simulink model "Control_test"  (R2014b)
settings: Solver=FixedStepDiscrete  StartTime=0.0  StopTime=Inf  FixedStep=0.001  RelTol=1e-3
PostLoadFcn:
  | , if any(exist('dsrtsu_mdlpostloadfcn', 'file') == [2, 3, 6]), try dsrtsu_mdlpostloadfcn('Execute', bdroot); catch fprintf('Error in PostLoadFcn (dsrtsu_mdlpostloadfcn) for model "%s":\n %s\n', bdroot, lasterr); end, end,
undefined symbols (not defined in the file or in its folder): dtLocal, slcm
libraries: rtican x163, simulink x14
(part 6 of 34)

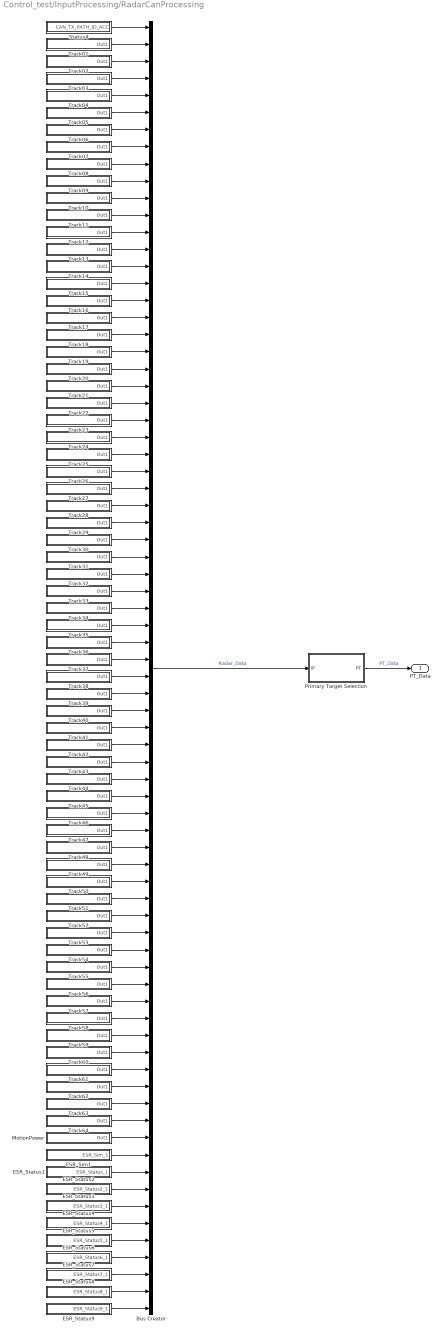
== system Control_test/InputProcessing/RadarCanProcessing ==
  Bus Creator : BusCreator  Inputs=76
  ESR_Sim1 : Subsystem
  ESR_Status1 : Subsystem
  ESR_Status2 : Subsystem
  ESR_Status3 : Subsystem
  ESR_Status4 : Subsystem
  ESR_Status5 : Subsystem
  ESR_Status6 : Subsystem
  ESR_Status7 : Subsystem
  ESR_Status8 : Subsystem
  ESR_Status9 : Subsystem
  MotionPower : Subsystem
  Primary Target Selection : Subsystem
  Status4 : Subsystem
  Track01 : Subsystem
  Track02 : Subsystem
  Track03 : Subsystem
  Track04 : Subsystem
  Track05 : Subsystem
  Track06 : Subsystem
  Track07 : Subsystem
  Track08 : Subsystem
  Track09 : Subsystem
  Track10 : Subsystem
  Track11 : Subsystem
  Track12 : Subsystem
  Track13 : Subsystem
  Track14 : Subsystem
  Track15 : Subsystem
  Track16 : Subsystem
  Track17 : Subsystem
  Track18 : Subsystem
  Track19 : Subsystem
  Track20 : Subsystem
  Track21 : Subsystem
  Track22 : Subsystem
  Track23 : Subsystem
  Track24 : Subsystem
  Track25 : Subsystem
  Track26 : Subsystem
  Track27 : Subsystem
  Track28 : Subsystem
  Track29 : Subsystem
  Track30 : Subsystem
  Track31 : Subsystem
  Track32 : Subsystem
  Track33 : Subsystem
  Track34 : Subsystem
  Track35 : Subsystem
  Track36 : Subsystem
  Track37 : Subsystem
  Track38 : Subsystem
  Track39 : Subsystem
  Track40 : Subsystem
  Track41 : Subsystem
  Track42 : Subsystem
  Track43 : Subsystem
  Track44 : Subsystem
  Track45 : Subsystem
  Track46 : Subsystem
  Track47 : Subsystem
  Track48 : Subsystem
  Track49 : Subsystem
  Track50 : Subsystem
  Track51 : Subsystem
  Track52 : Subsystem
  Track53 : Subsystem
  Track54 : Subsystem
  Track55 : Subsystem
  Track56 : Subsystem
  Track57 : Subsystem
  Track58 : Subsystem
  Track59 : Subsystem
  Track60 : Subsystem
  Track61 : Subsystem
  Track62 : Subsystem
  Track63 : Subsystem
  Track64 : Subsystem
  PT_Data : Outport
  wires:
  Status4/1(CAN_TX_PATH_ID_ACC) -> Bus Creator/1
  Track01/1(Out1) -> Bus Creator/2
  Track02/1(Out1) -> Bus Creator/3
  Track03/1(Out1) -> Bus Creator/4
  Track04/1(Out1) -> Bus Creator/5
  Track05/1(Out1) -> Bus Creator/6
  Track06/1(Out1) -> Bus Creator/7
  Track07/1(Out1) -> Bus Creator/8
  Track08/1(Out1) -> Bus Creator/9
  Track09/1(Out1) -> Bus Creator/10
  Track10/1(Out1) -> Bus Creator/11
  Track11/1(Out1) -> Bus Creator/12
  Track12/1(Out1) -> Bus Creator/13
  Track13/1(Out1) -> Bus Creator/14
  Track14/1(Out1) -> Bus Creator/15
  Track15/1(Out1) -> Bus Creator/16
  Track16/1(Out1) -> Bus Creator/17
  Track17/1(Out1) -> Bus Creator/18
  Track18/1(Out1) -> Bus Creator/19
  Track19/1(Out1) -> Bus Creator/20
  Track20/1(Out1) -> Bus Creator/21
  Track21/1(Out1) -> Bus Creator/22
  Track22/1(Out1) -> Bus Creator/23
  Track23/1(Out1) -> Bus Creator/24
  Track24/1(Out1) -> Bus Creator/25
  Track25/1(Out1) -> Bus Creator/26
  Track26/1(Out1) -> Bus Creator/27
  Track27/1(Out1) -> Bus Creator/28
  Track28/1(Out1) -> Bus Creator/29
  Track29/1(Out1) -> Bus Creator/30
  Track30/1(Out1) -> Bus Creator/31
  Track31/1(Out1) -> Bus Creator/32
  Track32/1(Out1) -> Bus Creator/33
  Track33/1(Out1) -> Bus Creator/34
  Track34/1(Out1) -> Bus Creator/35
  Track35/1(Out1) -> Bus Creator/36
  Track36/1(Out1) -> Bus Creator/37
  Track37/1(Out1) -> Bus Creator/38
  Track38/1(Out1) -> Bus Creator/39
  Track39/1(Out1) -> Bus Creator/40
  Track40/1(Out1) -> Bus Creator/41
  Track41/1(Out1) -> Bus Creator/42
  Track42/1(Out1) -> Bus Creator/43
  Track43/1(Out1) -> Bus Creator/44
  Track44/1(Out1) -> Bus Creator/45
  Track45/1(Out1) -> Bus Creator/46
  Track46/1(Out1) -> Bus Creator/47
  Track47/1(Out1) -> Bus Creator/48
  Track48/1(Out1) -> Bus Creator/49
  Track49/1(Out1) -> Bus Creator/50
  Track50/1(Out1) -> Bus Creator/51
  Track51/1(Out1) -> Bus Creator/52
  Track52/1(Out1) -> Bus Creator/53
  Track53/1(Out1) -> Bus Creator/54
  Track54/1(Out1) -> Bus Creator/55
  Track55/1(Out1) -> Bus Creator/56
  Track56/1(Out1) -> Bus Creator/57
  Track57/1(Out1) -> Bus Creator/58
  Track58/1(Out1) -> Bus Creator/59
  Track59/1(Out1) -> Bus Creator/60
  Track60/1(Out1) -> Bus Creator/61
  Track61/1(Out1) -> Bus Creator/62
  Track62/1(Out1) -> Bus Creator/63
  Track63/1(Out1) -> Bus Creator/64
  Track64/1(Out1) -> Bus Creator/65
  Bus Creator/1 -> Primary Target Selection/1(IP)  "Radar_Data"
  MotionPower/1(Out1) -> Bus Creator/66
  Primary Target Selection/1(PT) -> PT_Data/1  "PT_Data"
  ESR_Sim1/1(ESR_Sim_1) -> Bus Creator/67
  ESR_Status1/1(ESR_Status_1) -> Bus Creator/68
  ESR_Status2/1(ESR_Status2_1) -> Bus Creator/69
  ESR_Status3/1(ESR_Status3_1) -> Bus Creator/70
  ESR_Status4/1(ESR_Status4_1) -> Bus Creator/71
  ESR_Status5/1(ESR_Status5_1) -> Bus Creator/72
  ESR_Status6/1(ESR_Status6_1) -> Bus Creator/73
  ESR_Status7/1(ESR_Status7_1) -> Bus Creator/74
  ESR_Status8/1(ESR_Status8_1) -> Bus Creator/75
  ESR_Status9/1(ESR_Status9_1) -> Bus Creator/76

== system Control_test/InputProcessing/SensorFusion ==
  Bus Creator : BusCreator  Inputs=2
  Bus Creator1 : BusCreator  Inputs=2
  Bus Creator2 : BusCreator  Inputs=2
  Bus Creator3 : BusCreator  Inputs=3
  PTLeft_Data : rtican/RTICAN Receive (RX)   Reserved1=[]  Reserved2=[]  Reserved3=[]  Reserved4=[]  SfcnMessage=[]  Msg_Struct=[]  BoardTypeNo=[]  BoardNo=[]  ChannelNo=[]  Parameters=[]  DialogFcn=[]  UnitName=[]  Revision=[]  UnitValues=[]  DSProperties=struct('RTI',struct('Version',uint32(5),'BlockType',struct('isSLSource',uint8(1),'isSLSink',uint8(1),'isHWSource',uint8(0),'isHWSink',uint8(0),'isSetup',uint8(0),'isInline',uint8(1),'isNonInline',uint8(0),'isInterrupt',uint8(0),'isChannelwise',uint8(0)),'IOBoardType','RTICAN','UnitType','MESSAGE','Identifier','RX','DialogType','MSVC','BlockSet','RTICAN','SlaveProcessor','CAN'))  RTIBlockInterface=struct('OutputPortsWidth',int32([1 1]),'OutputPortsActive',[1 1],'OutputPortsName',{{'PTLeft_RelDist','PTLeft_RelSpeed'}},'OutputPortsDataType',{{'SS_DOUBLE','SS_DOUBLE'}},'OutputPortsLabel',{{'PTLeft_RelDist','PTLeft_RelSpeed'}},'OutputPortsLabelMode','ON','InputPortsWidth',int32(0),'InputPortsActive',0,'DialogFcn','rtican_message_interface_gui','BlockDisplay',{{'','center'}},'IconTransparency','on','ParameterTunableNames',{{}},'InitLevel',3,'BlockName',struct('Token',{{'PTLeft_Data'}}),'SampleTime',{{0.01}},'TriggerPort',{{'none'}},'EnablePort',{{'none'}})  RTIBlockParameters=struct('BoardTypeNo',{{1,'OFF',[]}},'BoardNo',{{2,'ON',[1 16]}},'ChannelNo',{{2,'ON',[1 2]}},'Parameters',{{struct('DataFileSupport',struct('DataFileSelectedMaster',1,'DataFileSelectedLocal',1,'DataFileName',['c:\users\mpc\documents\github\mpc-car\controller\dbcfiles\esr_dv3_64tgt.dbc|c:\users\mpc\dropbox\hyundai car setup\01_dbc_files\sensorfusion.dbc|'],'DataFileDate',['15-Dec-2015 14:58:47'],'SelectedFile',['..\..\..\..\..\..\dropbox\hyundai car setup\01_dbc_files\sensorfusion.dbc'],'InterfaceFcn','rtican_dbc_file_parser'),'Options',struct('StatusSelected',0,'TimeSelected',0,'DeltaTimeSelected',0,'BytePortSelected',0,'MessageLengthSelected',0,'TriggerPort',struct('Selected',0,'TriggerType',0),'UserCoding',struct('Selected',0,'InterfaceFile','UserDecodingFile','FcnName','UserDecodeFcn','InportSelected',0,'InportWidth',1,'OutportSelected',0,'OutportWidth',1),'EnablePortSelected',0,'SignalOnPortnameSelected',1,'UseRXService',0),'Message',struct('MsgOnBlocknameSelected',1,'MsgName','PTLeft_Data','MsgIdFormat',0,'MsgId',1585,'MsgLength',8,'NumSignals',2,'SampleTime',0.01,'Signal',struct('SgnName',{'PTLeft_RelDist','PTLeft_RelSpeed'},'SgnStartBit',{0,16},'SgnLength',{16,16},'SgnType',{0,0},'ModeValue',{-1,-1},'DataType',{1,1},'ByteLayout',{0,0},'Factor',{0.01,0.01},'Offset',{0,0},'SgnComment',{{''},{''}},'SgnUnit',{'m','m/s'},'Min',{-327.68,-327.68},'Max',{327.67,327.67},'SLDataType',{'SS_DOUBLE','SS_DOUBLE'}),'MsgIdNumFormat',0,'MsgComment',{{''}}),'Version',1.2,'general',struct('isFromLib',0)),'OFF',[]}},'GroupId',{{struct('Group',{{'RTICAN'}},'No',4,'Behavior',{{'NAMECHANGE'}},'BlockType',{{'SINK'}},'NameChangeFlag',0),'OFF',[]}},'SFcnRTICANMessage',{{struct('MsgType','RX','SFcnPortType','Scalar','MsgName','PTLeft_Data','MsgIdFormat','STD','MsgId',1585,'MsgLength',8,'NumSignals',2,'SampleTime',0.01,'Signal',struct('SgnName',{'PTLeft_RelDist','PTLeft_RelSpeed'},'SgnStartBit',{0,16},'SgnLength',{16,16},'SgnType',{'standard','standard'},'ModeValue',{-1,-1},'DataType',{['signed int'],['signed int']},'ByteLayout',{['little endian'],['little endian']},'Factor',{0.01,0.01},'Offset',{0,0},'SLDataType',{'SS_DOUBLE','SS_DOUBLE'}),'StatusSelected','no','TimeSelected','no','DeltaTimeSelected','no','BytePortSelected','no','MessageLengthSelected','no','TriggerPort',struct('Selected','no','TriggerType',0),'UserCoding',struct('Selected','no','InterfaceFile','UserDecodingFile','FcnName','UserDecodeFcn','InportSelected','no','InportWidth',1,'OutportSelected','no','OutportWidth',1),'EnablePortSelected','no','UseRXService','no','BoardType','DS1','BoardNo',2,'ControllerNo',2),'OFF',[]}},'TLCFileName',{{'rtican_rx_message','OFF',[]}})  RTISFcnParameters=struct('SFcnRTICANMessage','struct','TLCFileName','char')  RTIBlockParaDefault=struct('BoardTypeNo',4302,'BoardNo',1,'ChannelNo',1,'Parameters',struct('DataFileSupport',struct('DataFileSelectedMaster',0,'DataFileSelectedLocal',0,'DataFileName','','DataFileDate','','SelectedFile',['<no file selected>']),'Options',struct('StatusSelected',1,'TimeSelected',1,'DeltaTimeSelected',1,'BytePortSelected',0,'MessageLengthSelected',0,'TriggerPort',struct('Selected',0,'TriggerType','rising'),'UserCoding',struct('Selected',0,'InterfaceFile','UserDecodingFile','FcnName','UserDecodeFcn','InportSelected',0,'InportWidth',1,'OutportSelected',0,'OutportWidth',1),'EnablePortSelected',0,'SignalOnPortnameSelected',1,'UseRXService',0),'Message',struct('MsgOnBlocknameSelected',0,'MsgName',['RX Message'],'MsgIdFormat',0,'MsgId',100,'MsgLength',8,'NumSignals',1,'SampleTime',-1,'Signal',struct('SgnName',['RX signal'],'SgnStartBit',0,'SgnLength',8,'SgnType',0,'ModeValue',-1,'DataType',0,'SLDataType','SS_DOUBLE','ByteLayout',0,'Factor',1,'Offset',0,'Min',0,'Max',255,'SgnComment',{{}},'SgnUnit',''),'MsgIdNumFormat',0,'MsgComment',{{''}}),'Version',1.2,'general',struct('isFromLib',1)),'GroupId',struct('Group',{{'RTICAN'}},'No',1,'Behavior',{{'NAMECHANGE'}},'BlockType',{{'SINK'}},'NameChangeFlag',0),'SFcnRTICANMessage',struct('MsgType','RX','MsgName',['RX Message'],'MsgIdFormat','STD','MsgId',100,'MsgLength',8,'NumSignals',1,'SampleTime',-1,'Signal',struct('SgnName',['RX signal'],'SgnStartBit',0,'SgnLength',8,'SgnType','standard','ModeValue',-1,'DataType',['unsigned int'],'ByteLayout',['little endian'],'SLDataType','SS_DOUBLE','Factor',1,'Offset',0),'StatusSelected','yes','TimeSelected','yes','DeltaTimeSelected','yes','BytePortSelected','no','MessageLengthSelected','no','EnablePortSelected','no','UserCoding',struct('Selected','no','InterfaceFile','UserDecodingFile','FcnName','UserDecodeFcn','InportSelected','no','InportWidth',1,'OutportSelected','no','OutportWidth',1),'TriggerPort',struct('Selected','no','TriggerType','rising'),'UseRXService','no','BoardType','DS4302','BoardNo',1,'ControllerNo',1,'SFcnPortType','Scalar'),'TLCFileName','rtican_rx_message')
      settings: AttributesFormatString=Group Id: RTICAN4\n
  PTRight_Data : rtican/RTICAN Receive (RX)   Reserved1=[]  Reserved2=[]  Reserved3=[]  Reserved4=[]  SfcnMessage=[]  Msg_Struct=[]  BoardTypeNo=[]  BoardNo=[]  ChannelNo=[]  Parameters=[]  DialogFcn=[]  UnitName=[]  Revision=[]  UnitValues=[]  DSProperties=struct('RTI',struct('Version',uint32(5),'BlockType',struct('isSLSource',uint8(1),'isSLSink',uint8(1),'isHWSource',uint8(0),'isHWSink',uint8(0),'isSetup',uint8(0),'isInline',uint8(1),'isNonInline',uint8(0),'isInterrupt',uint8(0),'isChannelwise',uint8(0)),'IOBoardType','RTICAN','UnitType','MESSAGE','Identifier','RX','DialogType','MSVC','BlockSet','RTICAN','SlaveProcessor','CAN'))  RTIBlockInterface=struct('OutputPortsWidth',int32([1 1]),'OutputPortsActive',[1 1],'OutputPortsName',{{'PTRight_RelDist','PTRight_RelSpeed'}},'OutputPortsDataType',{{'SS_DOUBLE','SS_DOUBLE'}},'OutputPortsLabel',{{'PTRight_RelDist','PTRight_RelSpeed'}},'OutputPortsLabelMode','ON','InputPortsWidth',int32(0),'InputPortsActive',0,'DialogFcn','rtican_message_interface_gui','BlockDisplay',{{'','center'}},'IconTransparency','on','ParameterTunableNames',{{}},'InitLevel',3,'BlockName',struct('Token',{{'PTRight_Data'}}),'SampleTime',{{0.01}},'TriggerPort',{{'none'}},'EnablePort',{{'none'}})  RTIBlockParameters=struct('BoardTypeNo',{{1,'OFF',[]}},'BoardNo',{{2,'ON',[1 16]}},'ChannelNo',{{2,'ON',[1 2]}},'Parameters',{{struct('DataFileSupport',struct('DataFileSelectedMaster',1,'DataFileSelectedLocal',1,'DataFileName',['c:\users\mpc\documents\github\mpc-car\controller\dbcfiles\esr_dv3_64tgt.dbc|c:\users\mpc\dropbox\hyundai car setup\01_dbc_files\sensorfusion.dbc|'],'DataFileDate',['15-Dec-2015 14:58:47'],'SelectedFile',['..\..\..\..\..\..\dropbox\hyundai car setup\01_dbc_files\sensorfusion.dbc'],'InterfaceFcn','rtican_dbc_file_parser'),'Options',struct('StatusSelected',0,'TimeSelected',0,'DeltaTimeSelected',0,'BytePortSelected',0,'MessageLengthSelected',0,'TriggerPort',struct('Selected',0,'TriggerType',0),'UserCoding',struct('Selected',0,'InterfaceFile','UserDecodingFile','FcnName','UserDecodeFcn','InportSelected',0,'InportWidth',1,'OutportSelected',0,'OutportWidth',1),'EnablePortSelected',0,'SignalOnPortnameSelected',1,'UseRXService',0),'Message',struct('MsgOnBlocknameSelected',1,'MsgName','PTRight_Data','MsgIdFormat',0,'MsgId',1586,'MsgLength',8,'NumSignals',2,'SampleTime',0.01,'Signal',struct('SgnName',{'PTRight_RelDist','PTRight_RelSpeed'},'SgnStartBit',{0,16},'SgnLength',{16,16},'SgnType',{0,0},'ModeValue',{-1,-1},'DataType',{1,1},'ByteLayout',{0,0},'Factor',{0.01,0.01},'Offset',{0,0},'SgnComment',{{''},{''}},'SgnUnit',{'m','m/s'},'Min',{-327.68,-327.68},'Max',{327.67,327.67},'SLDataType',{'SS_DOUBLE','SS_DOUBLE'}),'MsgIdNumFormat',0,'MsgComment',{{''}}),'Version',1.2,'general',struct('isFromLib',0)),'OFF',[]}},'GroupId',{{struct('Group',{{'RTICAN'}},'No',4,'Behavior',{{'NAMECHANGE'}},'BlockType',{{'SINK'}},'NameChangeFlag',0),'OFF',[]}},'SFcnRTICANMessage',{{struct('MsgType','RX','SFcnPortType','Scalar','MsgName','PTRight_Data','MsgIdFormat','STD','MsgId',1586,'MsgLength',8,'NumSignals',2,'SampleTime',0.01,'Signal',struct('SgnName',{'PTRight_RelDist','PTRight_RelSpeed'},'SgnStartBit',{0,16},'SgnLength',{16,16},'SgnType',{'standard','standard'},'ModeValue',{-1,-1},'DataType',{['signed int'],['signed int']},'ByteLayout',{['little endian'],['little endian']},'Factor',{0.01,0.01},'Offset',{0,0},'SLDataType',{'SS_DOUBLE','SS_DOUBLE'}),'StatusSelected','no','TimeSelected','no','DeltaTimeSelected','no','BytePortSelected','no','MessageLengthSelected','no','TriggerPort',struct('Selected','no','TriggerType',0),'UserCoding',struct('Selected','no','InterfaceFile','UserDecodingFile','FcnName','UserDecodeFcn','InportSelected','no','InportWidth',1,'OutportSelected','no','OutportWidth',1),'EnablePortSelected','no','UseRXService','no','BoardType','DS1','BoardNo',2,'ControllerNo',2),'OFF',[]}},'TLCFileName',{{'rtican_rx_message','OFF',[]}})  RTISFcnParameters=struct('SFcnRTICANMessage','struct','TLCFileName','char')  RTIBlockParaDefault=struct('BoardTypeNo',4302,'BoardNo',1,'ChannelNo',1,'Parameters',struct('DataFileSupport',struct('DataFileSelectedMaster',0,'DataFileSelectedLocal',0,'DataFileName','','DataFileDate','','SelectedFile',['<no file selected>']),'Options',struct('StatusSelected',1,'TimeSelected',1,'DeltaTimeSelected',1,'BytePortSelected',0,'MessageLengthSelected',0,'TriggerPort',struct('Selected',0,'TriggerType','rising'),'UserCoding',struct('Selected',0,'InterfaceFile','UserDecodingFile','FcnName','UserDecodeFcn','InportSelected',0,'InportWidth',1,'OutportSelected',0,'OutportWidth',1),'EnablePortSelected',0,'SignalOnPortnameSelected',1,'UseRXService',0),'Message',struct('MsgOnBlocknameSelected',0,'MsgName',['RX Message'],'MsgIdFormat',0,'MsgId',100,'MsgLength',8,'NumSignals',1,'SampleTime',-1,'Signal',struct('SgnName',['RX signal'],'SgnStartBit',0,'SgnLength',8,'SgnType',0,'ModeValue',-1,'DataType',0,'SLDataType','SS_DOUBLE','ByteLayout',0,'Factor',1,'Offset',0,'Min',0,'Max',255,'SgnComment',{{}},'SgnUnit',''),'MsgIdNumFormat',0,'MsgComment',{{''}}),'Version',1.2,'general',struct('isFromLib',1)),'GroupId',struct('Group',{{'RTICAN'}},'No',1,'Behavior',{{'NAMECHANGE'}},'BlockType',{{'SINK'}},'NameChangeFlag',0),'SFcnRTICANMessage',struct('MsgType','RX','MsgName',['RX Message'],'MsgIdFormat','STD','MsgId',100,'MsgLength',8,'NumSignals',1,'SampleTime',-1,'Signal',struct('SgnName',['RX signal'],'SgnStartBit',0,'SgnLength',8,'SgnType','standard','ModeValue',-1,'DataType',['unsigned int'],'ByteLayout',['little endian'],'SLDataType','SS_DOUBLE','Factor',1,'Offset',0),'StatusSelected','yes','TimeSelected','yes','DeltaTimeSelected','yes','BytePortSelected','no','MessageLengthSelected','no','EnablePortSelected','no','UserCoding',struct('Selected','no','InterfaceFile','UserDecodingFile','FcnName','UserDecodeFcn','InportSelected','no','InportWidth',1,'OutportSelected','no','OutportWidth',1),'TriggerPort',struct('Selected','no','TriggerType','rising'),'UseRXService','no','BoardType','DS4302','BoardNo',1,'ControllerNo',1,'SFcnPortType','Scalar'),'TLCFileName','rtican_rx_message')
      settings: AttributesFormatString=Group Id: RTICAN4\n
  PT_Data : rtican/RTICAN Receive (RX)   Reserved1=[]  Reserved2=[]  Reserved3=[]  Reserved4=[]  SfcnMessage=[]  Msg_Struct=[]  BoardTypeNo=[]  BoardNo=[]  ChannelNo=[]  Parameters=[]  DialogFcn=[]  UnitName=[]  Revision=[]  UnitValues=[]  DSProperties=struct('RTI',struct('Version',uint32(5),'BlockType',struct('isSLSource',uint8(1),'isSLSink',uint8(1),'isHWSource',uint8(0),'isHWSink',uint8(0),'isSetup',uint8(0),'isInline',uint8(1),'isNonInline',uint8(0),'isInterrupt',uint8(0),'isChannelwise',uint8(0)),'IOBoardType','RTICAN','UnitType','MESSAGE','Identifier','RX','DialogType','MSVC','BlockSet','RTICAN','SlaveProcessor','CAN'))  RTIBlockInterface=struct('OutputPortsWidth',int32([1 1]),'OutputPortsActive',[1 1],'OutputPortsName',{{'PT_RelDist','PT_RelSpeed'}},'OutputPortsDataType',{{'SS_DOUBLE','SS_DOUBLE'}},'OutputPortsLabel',{{'PT_RelDist','PT_RelSpeed'}},'OutputPortsLabelMode','ON','InputPortsWidth',int32(0),'InputPortsActive',0,'DialogFcn','rtican_message_interface_gui','BlockDisplay',{{'','center'}},'IconTransparency','on','ParameterTunableNames',{{}},'InitLevel',3,'BlockName',struct('Token',{{'PT_Data'}}),'SampleTime',{{0.01}},'TriggerPort',{{'none'}},'EnablePort',{{'none'}})  RTIBlockParameters=struct('BoardTypeNo',{{1,'OFF',[]}},'BoardNo',{{2,'ON',[1 16]}},'ChannelNo',{{2,'ON',[1 2]}},'Parameters',{{struct('DataFileSupport',struct('DataFileSelectedMaster',1,'DataFileSelectedLocal',1,'DataFileName',['c:\users\mpc\documents\github\mpc-car\controller\dbcfiles\esr_dv3_64tgt.dbc|c:\users\mpc\dropbox\hyundai car setup\01_dbc_files\sensorfusion.dbc|'],'DataFileDate',['15-Dec-2015 14:58:47'],'SelectedFile',['..\..\..\..\..\..\dropbox\hyundai car setup\01_dbc_files\sensorfusion.dbc'],'InterfaceFcn','rtican_dbc_file_parser'),'Options',struct('StatusSelected',0,'TimeSelected',0,'DeltaTimeSelected',0,'BytePortSelected',0,'MessageLengthSelected',0,'TriggerPort',struct('Selected',0,'TriggerType',0),'UserCoding',struct('Selected',0,'InterfaceFile','UserDecodingFile','FcnName','UserDecodeFcn','InportSelected',0,'InportWidth',1,'OutportSelected',0,'OutportWidth',1),'EnablePortSelected',0,'SignalOnPortnameSelected',1,'UseRXService',0),'Message',struct('MsgOnBlocknameSelected',1,'MsgName','PT_Data','MsgIdFormat',0,'MsgId',1584,'MsgLength',8,'NumSignals',2,'SampleTime',0.01,'Signal',struct('SgnName',{'PT_RelDist','PT_RelSpeed'},'SgnStartBit',{0,16},'SgnLength',{16,16},'SgnType',{0,0},'ModeValue',{-1,-1},'DataType',{1,1},'ByteLayout',{0,0},'Factor',{0.01,0.01},'Offset',{0,0},'SgnComment',{{''},{''}},'SgnUnit',{'m','m/s'},'Min',{-327.68,-327.68},'Max',{327.67,327.67},'SLDataType',{'SS_DOUBLE','SS_DOUBLE'}),'MsgIdNumFormat',0,'MsgComment',{{''}}),'Version',1.2,'general',struct('isFromLib',0)),'OFF',[]}},'GroupId',{{struct('Group',{{'RTICAN'}},'No',4,'Behavior',{{'NAMECHANGE'}},'BlockType',{{'SINK'}},'NameChangeFlag',0),'OFF',[]}},'SFcnRTICANMessage',{{struct('MsgType','RX','SFcnPortType','Scalar','MsgName','PT_Data','MsgIdFormat','STD','MsgId',1584,'MsgLength',8,'NumSignals',2,'SampleTime',0.01,'Signal',struct('SgnName',{'PT_RelDist','PT_RelSpeed'},'SgnStartBit',{0,16},'SgnLength',{16,16},'SgnType',{'standard','standard'},'ModeValue',{-1,-1},'DataType',{['signed int'],['signed int']},'ByteLayout',{['little endian'],['little endian']},'Factor',{0.01,0.01},'Offset',{0,0},'SLDataType',{'SS_DOUBLE','SS_DOUBLE'}),'StatusSelected','no','TimeSelected','no','DeltaTimeSelected','no','BytePortSelected','no','MessageLengthSelected','no','TriggerPort',struct('Selected','no','TriggerType',0),'UserCoding',struct('Selected','no','InterfaceFile','UserDecodingFile','FcnName','UserDecodeFcn','InportSelected','no','InportWidth',1,'OutportSelected','no','OutportWidth',1),'EnablePortSelected','no','UseRXService','no','BoardType','DS1','BoardNo',2,'ControllerNo',2),'OFF',[]}},'TLCFileName',{{'rtican_rx_message','OFF',[]}})  RTISFcnParameters=struct('SFcnRTICANMessage','struct','TLCFileName','char')  RTIBlockParaDefault=struct('BoardTypeNo',4302,'BoardNo',1,'ChannelNo',1,'Parameters',struct('DataFileSupport',struct('DataFileSelectedMaster',0,'DataFileSelectedLocal',0,'DataFileName','','DataFileDate','','SelectedFile',['<no file selected>']),'Options',struct('StatusSelected',1,'TimeSelected',1,'DeltaTimeSelected',1,'BytePortSelected',0,'MessageLengthSelected',0,'TriggerPort',struct('Selected',0,'TriggerType','rising'),'UserCoding',struct('Selected',0,'InterfaceFile','UserDecodingFile','FcnName','UserDecodeFcn','InportSelected',0,'InportWidth',1,'OutportSelected',0,'OutportWidth',1),'EnablePortSelected',0,'SignalOnPortnameSelected',1,'UseRXService',0),'Message',struct('MsgOnBlocknameSelected',0,'MsgName',['RX Message'],'MsgIdFormat',0,'MsgId',100,'MsgLength',8,'NumSignals',1,'SampleTime',-1,'Signal',struct('SgnName',['RX signal'],'SgnStartBit',0,'SgnLength',8,'SgnType',0,'ModeValue',-1,'DataType',0,'SLDataType','SS_DOUBLE','ByteLayout',0,'Factor',1,'Offset',0,'Min',0,'Max',255,'SgnComment',{{}},'SgnUnit',''),'MsgIdNumFormat',0,'MsgComment',{{''}}),'Version',1.2,'general',struct('isFromLib',1)),'GroupId',struct('Group',{{'RTICAN'}},'No',1,'Behavior',{{'NAMECHANGE'}},'BlockType',{{'SINK'}},'NameChangeFlag',0),'SFcnRTICANMessage',struct('MsgType','RX','MsgName',['RX Message'],'MsgIdFormat','STD','MsgId',100,'MsgLength',8,'NumSignals',1,'SampleTime',-1,'Signal',struct('SgnName',['RX signal'],'SgnStartBit',0,'SgnLength',8,'SgnType','standard','ModeValue',-1,'DataType',['unsigned int'],'ByteLayout',['little endian'],'SLDataType','SS_DOUBLE','Factor',1,'Offset',0),'StatusSelected','yes','TimeSelected','yes','DeltaTimeSelected','yes','BytePortSelected','no','MessageLengthSelected','no','EnablePortSelected','no','UserCoding',struct('Selected','no','InterfaceFile','UserDecodingFile','FcnName','UserDecodeFcn','InportSelected','no','InportWidth',1,'OutportSelected','no','OutportWidth',1),'TriggerPort',struct('Selected','no','TriggerType','rising'),'UseRXService','no','BoardType','DS4302','BoardNo',1,'ControllerNo',1,'SFcnPortType','Scalar'),'TLCFileName','rtican_rx_message')
      settings: AttributesFormatString=Group Id: RTICAN4\n
  PTDataFusion : Outport
  wires:
  Bus Creator3/1 -> PTDataFusion/1  "PTDataFusion"
  Bus Creator/1 -> Bus Creator3/1  "PT_Data"
  Bus Creator1/1 -> Bus Creator3/2  "PTLeft_Data"
  Bus Creator2/1 -> Bus Creator3/3  "PTRight_Data"
  PT_Data/1 -> Bus Creator/1  "PT_RelDist"
  PT_Data/2 -> Bus Creator/2  "PT_RelSpeed"
  PTLeft_Data/1 -> Bus Creator1/1  "PTLeft_RelDist"
  PTLeft_Data/2 -> Bus Creator1/2  "PTLeft_RelSpeed"
  PTRight_Data/1 -> Bus Creator2/1  "PTRight_RelDist"
  PTRight_Data/2 -> Bus Creator2/2  "PTRight_RelSpeed"

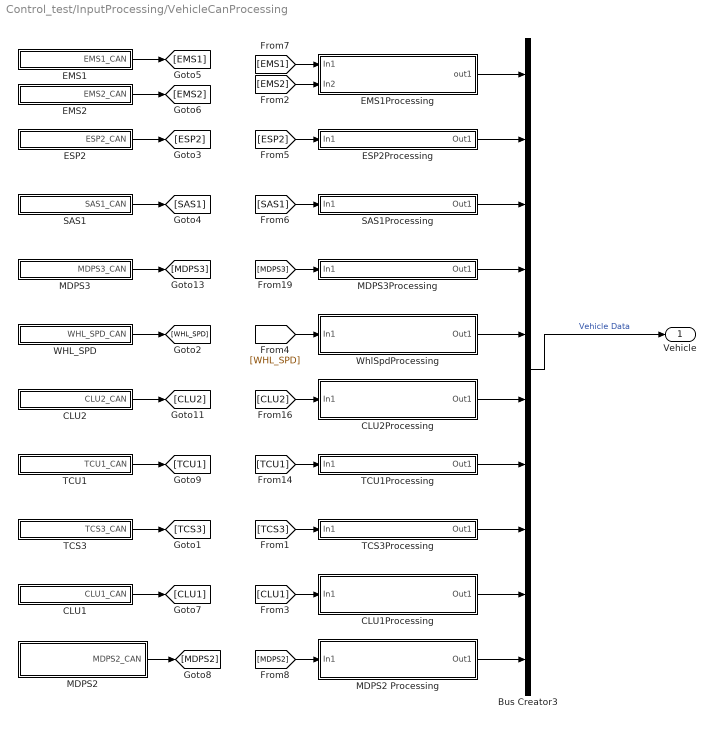
== system Control_test/InputProcessing/VehicleCanProcessing ==
  Bus Creator3 : BusCreator  Inputs=10
  CLU1 : Subsystem
  CLU1Processing : Subsystem
  CLU2 : Subsystem
  CLU2Processing : Subsystem
  EMS1 : Subsystem
  EMS1Processing : Subsystem
  EMS2 : Subsystem
  ESP2 : Subsystem
  ESP2Processing : Subsystem
  MDPS2 : Subsystem
  MDPS2 Processing : Subsystem
  MDPS3 : Subsystem
  MDPS3Processing : Subsystem
  SAS1 : Subsystem
  SAS1Processing : Subsystem
  TCS3 : Subsystem
  TCS3Processing : Subsystem
  TCU1 : Subsystem
  TCU1Processing : Subsystem
  WHL_SPD : Subsystem
  WhlSpdProcessing : Subsystem
  Vehicle : Outport
  wires:
  WHL_SPD/1(WHL_SPD_CAN) -> [WHL_SPD]
  ESP2/1(ESP2_CAN) -> [ESP2]
  SAS1/1(SAS1_CAN) -> [SAS1]
  CLU2/1(CLU2_CAN) -> [CLU2]
  [WHL_SPD] -> WhlSpdProcessing/1(In1)
  [SAS1] -> SAS1Processing/1(In1)
  [CLU2] -> CLU2Processing/1(In1)
  MDPS3/1(MDPS3_CAN) -> [MDPS3]
  [MDPS3] -> MDPS3Processing/1(In1)
  [EMS1] -> EMS1Processing/1(In1)
  [ESP2] -> ESP2Processing/1(In1)
  EMS1Processing/1(out1) -> Bus Creator3/1
  TCU1/1(TCU1_CAN) -> [TCU1]
  [TCU1] -> TCU1Processing/1(In1)
  Bus Creator3/1 -> Vehicle/1  "Vehicle Data"
  EMS1/1(EMS1_CAN) -> [EMS1]
  EMS2/1(EMS2_CAN) -> [EMS2]
  [EMS2] -> EMS1Processing/2(In2)
  ESP2Processing/1(Out1) -> Bus Creator3/2
  SAS1Processing/1(Out1) -> Bus Creator3/3
  MDPS3Processing/1(Out1) -> Bus Creator3/4
  WhlSpdProcessing/1(Out1) -> Bus Creator3/5
  CLU2Processing/1(Out1) -> Bus Creator3/6
  TCU1Processing/1(Out1) -> Bus Creator3/7
  TCS3/1(TCS3_CAN) -> [TCS3]
  [TCS3] -> TCS3Processing/1(In1)
  TCS3Processing/1(Out1) -> Bus Creator3/8
  CLU1/1(CLU1_CAN) -> [CLU1]
  [CLU1] -> CLU1Processing/1(In1)
  CLU1Processing/1(Out1) -> Bus Creator3/9
  MDPS2/1(MDPS2_CAN) -> [MDPS2]
  [MDPS2] -> MDPS2 Processing/1(In1)
  MDPS2 Processing/1(Out1) -> Bus Creator3/10

== system Control_test/OutputProcessing/ACC_Interface ==
  note: 0 : OFF
      | 1: STANDBY
      | 2: CONTROL
      | 3 : STOP
      | 4 : HOLD
      | 5 : OVERRIDE
      | 6 : SHUTDOWN
  aReq : Inport
  DriverOverride_flag : Inport  Port=2
  Clearance : Constant  Value=255
  Headway : Constant  Value=4
  L_SCC1 : rtican/RTICAN Transmit (TX)   Reserved1=[]  Reserved2=[]  Reserved3=[]  Reserved4=[]  SfcnMessage=[]  Msg_Struct=[]  BoardTypeNo=[]  BoardNo=[]  ChannelNo=[]  Parameters=[]  DialogFcn=[]  UnitName=[]  Revision=[]  UnitValues=[]  DSProperties=struct('RTI',struct('Version',uint32(5),'BlockType',struct('isSLSource',uint8(1),'isSLSink',uint8(1),'isHWSource',uint8(0),'isHWSink',uint8(0),'isSetup',uint8(0),'isInline',uint8(1),'isNonInline',uint8(0),'isInterrupt',uint8(0),'isChannelwise',uint8(0)),'IOBoardType','RTICAN','UnitType','MESSAGE','Identifier','TX','DialogType','MSVC','BlockSet','RTICAN','SlaveProcessor','CAN'))  RTIBlockInterface=struct('InputPortsWidth',int32([1 1 1 1 1 1 1 1 1 1 1 1 1 1]),'InputPortsActive',[1 1 1 1 1 1 1 1 1 1 1 1 1 1],'InputPortsName',{{'aReqMax','MainMode_ACC','AliveCounterACC','aReqMin','VSetDis','SCCInfoDisplay','ACCFailInfo','ACCMode','StopReq','PreFill','ObjValid','TakeOverReq','TauGapSet','DriverAlertDisplay'}},'InputPortsDataType',{{'SS_DOUBLE','SS_DOUBLE','SS_DOUBLE','SS_DOUBLE','SS_DOUBLE','SS_DOUBLE','SS_DOUBLE','SS_DOUBLE','SS_DOUBLE','SS_DOUBLE','SS_DOUBLE','SS_DOUBLE','SS_DOUBLE','SS_DOUBLE'}},'OutputPortsWidth',int32(0),'OutputPortsActive',0,'OutputPortsName',{{''}},'DialogFcn','rtican_message_interface_gui','BlockDisplay',{{'','center'}},'IconTransparency','on','InitLevel',3,'BlockName',struct('Token',{{'L_SCC1'}}),'SampleTime',{{0.02}},'TriggerPort',{{'none'}},'EnablePort',{{'none'}})  RTIBlockParameters=struct('BoardTypeNo',{{1,'OFF',[]}},'BoardNo',{{1,'ON',[1 16]}},'ChannelNo',{{1,'ON',[1 2]}},'Parameters',{{struct('DataFileSupport',struct('DataFileSelectedMaster',1,'DataFileSelectedLocal',1,'DataFileName',['c:\users\mpc\dropbox\hyundai car setup\hmc_can_for_ucb_v1.dbc|c:\users\mpc\dropbox\hyundai car setup\mobileye spec new\mobileye_mando_camera_ucb_v2.dbc|'],'DataFileDate',['26-Nov-2014 10:54:28'],'SelectedFile','c:\users\mpc_car\documents\github\mpc-car\dbcfiles\hmc_can_for_ucb_v2.dbc','InterfaceFcn','rtican_dbc_file_parser'),'Options',struct('StatusSelected',0,'TimeSelected',0,'DeltaTimeSelected',0,'DelayTimeSelected',0,'DelayTimeTXCommandSelected',0,'EncodeSetUnusedBitsToOne',0,'EnableMsgLoopback',0,'TriggerPort',struct('Selected',0,'TriggerType',0),'EnablePortSelected',0,'SignalOnPortnameSelected',1,'UserCoding',struct('Selected',0,'InterfaceFile','UserEncodingFile','FcnName','UserEncodeFcn','InportSelected',0,'InportWidth',1,'OutportSelected',0,'OutportWidth',1),'TerminationMsg',struct('Selected',0,'Byte0_7','0'),'InitialMsg',struct('Selected',0,'Byte0_7','0')),'Message',struct('MsgOnBlocknameSelected',1,'MsgName','L_SCC1','MsgIdFormat',0,'MsgId',256,'MsgLength',8,'NumSignals',14,'SampleTime',0.02,'StartTime',struct('Selected',0,'Value',0),'AutoRepeatTime',struct('Selected',0,'Value',0.1),'Timeout',struct('Selected',0,'Value',0.1),'DelayTime',struct('Selected',0,'Value',0.1),'Signal',struct('SgnName',{'aReqMax','MainMode_ACC','AliveCounterACC','aReqMin','VSetDis','SCCInfoDisplay','ACCFailInfo','ACCMode','StopReq','PreFill','ObjValid','TakeOverReq','TauGapSet','DriverAlertDisplay'},'SgnStartBit',{0,11,12,16,40,48,51,53,55,56,57,58,59,62},'SgnLength',{11,1,4,11,8,3,2,2,1,1,1,1,3,2},'ByteLayout',{0,0,0,0,0,0,0,0,0,0,0,0,0,0},'Factor',{0.01,1,1,0.01,1,1,1,1,1,1,1,1,1,1},'Offset',{-10.23,0,0,-10.23,0,0,0,0,0,0,0,0,0,0},'SgnComment',{'','','','',['This signal can be sent in km/h or MPH according to the ¡°SPEED_UNIT¡± signal (See CLU1 message).'],'','','','','','','','',''},'SgnUnit',{'m/s^2','','','m/s^2',['km/h or MPH'],'','','','','','','','',''},'Min',{-10.23,0,0,-10.23,0,0,0,0,0,0,0,0,0,0},'Max',{10.24,1,15,10.24,255,7,3,3,1,1,1,1,7,3},'SgnType',{0,0,0,0,0,0,0,0,0,0,0,0,0,0},'SLDataType',{'SS_DOUBLE','SS_DOUBLE','SS_DOUBLE','SS_DOUBLE','SS_DOUBLE','SS_DOUBLE','SS_DOUBLE','SS_DOUBLE','SS_DOUBLE','SS_DOUBLE','SS_DOUBLE','SS_DOUBLE','SS_DOUBLE','SS_DOUBLE'},'DataType',{0,0,0,0,0,0,0,0,0,0,0,0,0,0},'ModeValue',{-1,-1,-1,-1,-1,-1,-1,-1,-1,-1,-1,-1,-1,-1}),'MsgIdNumFormat',0,'MsgComment',{{''}}),'Version',1.2,'general',struct('isFromLib',0)),'OFF',[]}},'GroupId',{{struct('Group',{{'RTICAN'}},'No',1,'Behavior',{{'NAMECHANGE'}},'BlockType',{{'SINK'}},'NameChangeFlag',0),'OFF',[]}},'SFcnRTICANMessage',{{struct('MsgType','TX','SFcnPortType','Scalar','MsgName','L_SCC1','MsgIdFormat','STD','MsgId',256,'MsgLength',8,'NumSignals',14,'SampleTime',0.02,'StartTime',struct('Selected','no','Value',0),'AutoRepeatTime',struct('Selected','no','Value',0.1),'Timeout',struct('Selected','no','Value',0.1),'Signal',struct('SgnName',{'aReqMax','MainMode_ACC','AliveCounterACC','aReqMin','VSetDis','SCCInfoDisplay','ACCFailInfo','ACCMode','StopReq','PreFill','ObjValid','TakeOverReq','TauGapSet','DriverAlertDisplay'},'SgnStartBit',{0,11,12,16,40,48,51,53,55,56,57,58,59,62},'SgnLength',{11,1,4,11,8,3,2,2,1,1,1,1,3,2},'ByteLayout',{['little endian'],['little endian'],['little endian'],['little endian'],['little endian'],['little endian'],['little endian'],['little endian'],['little endian'],['little endian'],['little endian'],['little endian'],['little endian'],['little endian']},'Factor',{0.01,1,1,0.01,1,1,1,1,1,1,1,1,1,1},'Offset',{-10.23,0,0,-10.23,0,0,0,0,0,0,0,0,0,0},'SgnType',{'standard','standard','standard','standard','standard','standard','standard','standard','standard','standard','standard','standard','standard','standard'},'SLDataType',{'SS_DOUBLE','SS_DOUBLE','SS_DOUBLE','SS_DOUBLE','SS_DOUBLE','SS_DOUBLE','SS_DOUBLE','SS_DOUBLE','SS_DOUBLE','SS_DOUBLE','SS_DOUBLE','SS_DOUBLE','SS_DOUBLE','SS_DOUBLE'},'DataType',{['unsigned int'],['unsigned int'],['unsigned int'],['unsigned int'],['unsigned int'],['unsigned int'],['unsigned int'],['unsigned int'],['unsigned int'],['unsigned int'],['unsigned int'],['unsigned int'],['unsigned int'],['unsigned int']},'ModeValue',{-1,-1,-1,-1,-1,-1,-1,-1,-1,-1,-1,-1,-1,-1}),'StatusSelected','no','TimeSelected','no','DeltaTimeSelected','no','DelayTimeSelected','no','DelayTimeTXCommandSelected','no','EncodeSetUnusedBitsToOne','no','EnableMsgLoopback','no','TriggerPort',struct('Selected','no','TriggerType',0),'EnablePortSelected','no','UserCoding',struct('Selected','no','InterfaceFile','UserEncodingFile','FcnName','UserEncodeFcn','InportSelected','no','InportWidth',1,'OutportSelected','no','OutportWidth',1),'TerminationMsg',struct('Selected','no','Byte0','0x00','Byte1','0x00','Byte2','0x00','Byte3','0x00','Byte4','0x00','Byte5','0x00','Byte6','0x00','Byte7','0x00'),'InitialMsg',struct('Selected','no','Byte0','0x00','Byte1','0x00','Byte2','0x00','Byte3','0x00','Byte4','0x00','Byte5','0x00','Byte6','0x00','Byte7','0x00'),'BoardType','DS1','BoardNo',1,'ControllerNo',1),'OFF',[]}},'TLCFileName',{{'rtican_tx_message','OFF',[]}})  RTISFcnParameters=struct('SFcnRTICANMessage','struct','TLCFileName','char')  RTIBlockParaDefault=struct('BoardTypeNo',4302,'BoardNo',1,'ChannelNo',1,'Parameters',struct('DataFileSupport',struct('DataFileSelectedMaster',0,'DataFileSelectedLocal',0,'DataFileName','','DataFileDate','','SelectedFile',['<no file selected>']),'Options',struct('StatusSelected',1,'TimeSelected',1,'DeltaTimeSelected',1,'DelayTimeSelected',1,'DelayTimeTXCommandSelected',0,'EncodeSetUnusedBitsToOne',0,'EnableMsgLoopback',0,'TriggerPort',struct('Selected',0,'TriggerType','rising'),'EnablePortSelected',0,'SignalOnPortnameSelected',1,'UserCoding',struct('Selected',0,'InterfaceFile','UserEncodingFile','FcnName','UserEncodeFcn','InportSelected',0,'InportWidth',1,'OutportSelected',0,'OutportWidth',1),'TerminationMsg',struct('Selected',0,'Byte0_7','0'),'InitialMsg',struct('Selected',0,'Byte0_7','0')),'Message',struct('MsgOnBlocknameSelected',0,'MsgName',['TX Message'],'MsgIdFormat',0,'MsgId',100,'MsgLength',8,'NumSignals',1,'SampleTime',-1,'StartTime',struct('Selected',0,'Value',0),'AutoRepeatTime',struct('Selected',0,'Value',0.1),'Timeout',struct('Selected',0,'Value',0.1),'DelayTime',struct('Selected',0,'Value',0.1),'Signal',struct('SgnName',['TX signal'],'SgnStartBit',0,'SgnLength',8,'SgnType',0,'ModeValue',-1,'DataType',0,'SLDataType','SS_DOUBLE','ByteLayout',0,'Factor',1,'Offset',0,'Min',0,'Max',255,'SgnComment',{{}},'SgnUnit',''),'MsgIdNumFormat',0,'MsgComment',{{''}}),'Version',1.2,'general',struct('isFromLib',1)),'GroupId',struct('Group',{{'RTICAN'}},'No',1,'Behavior',{{'NAMECHANGE'}},'BlockType',{{'SINK'}},'NameChangeFlag',0),'SFcnRTICANMessage',struct('MsgType','TX','MsgName',['TX Message'],'MsgIdFormat','STD','MsgId',100,'MsgLength',2,'NumSignals',1,'SampleTime',-1,'StartTime',struct('Selected','no','Value',0),'AutoRepeatTime',struct('Selected','no','Value',0.1),'Timeout',struct('Selected','no','Value',0.1),'DelayTime',struct('Selected','no','Value',0.1),'Signal',struct('SgnName',['TX signal'],'SgnStartBit',0,'SgnLength',8,'SgnType','standard','ModeValue',-1,'DataType',['unsigned int'],'ByteLayout',['little endian'],'SLDataType','SS_DOUBLE','Factor',1,'Offset',0),'StatusSelected','yes','TimeSelected','yes','DeltaTimeSelected','yes','DelayTimeSelected','yes','EnablePortSelected','no','EnableMsgLoopback','no','DelayTimeTXCommandSelected','no','EncodeSetUnusedBitsToOne','no','UserCoding',struct('Selected','no','InterfaceFile','UserDecodingFile','FcnName','UserDecodeFcn','InportSelected','no','InportWidth',1,'OutportSelected','no','OutportWidth',1),'TerminationMsg',struct('Selected','no','Byte0','0x00','Byte1','0x00','Byte2','0x00','Byte3','0x00','Byte4','0x00','Byte5','0x00','Byte6','0x00','Byte7','0x00'),'InitialMsg',struct('Selected','no','Byte0','0x00','Byte1','0x00','Byte2','0x00','Byte3','0x00','Byte4','0x00','Byte5','0x00','Byte6','0x00','Byte7','0x00'),'TriggerPort',struct('Selected','no','TriggerType','rising'),'BoardType','DS4302','BoardNo',1,'ControllerNo',1,'SFcnPortType','Scalar'),'TLCFileName','rtican_tx_message')
      settings: AttributesFormatString=Group Id: RTICAN1\n
  L_SCC2 : rtican/RTICAN Transmit (TX)   Reserved1=[]  Reserved2=[]  Reserved3=[]  Reserved4=[]  SfcnMessage=[]  Msg_Struct=[]  BoardTypeNo=[]  BoardNo=[]  ChannelNo=[]  Parameters=[]  DialogFcn=[]  UnitName=[]  Revision=[]  UnitValues=[]  DSProperties=struct('RTI',struct('Version',uint32(5),'BlockType',struct('isSLSource',uint8(1),'isSLSink',uint8(1),'isHWSource',uint8(0),'isHWSink',uint8(0),'isSetup',uint8(0),'isInline',uint8(1),'isNonInline',uint8(0),'isInterrupt',uint8(0),'isChannelwise',uint8(0)),'IOBoardType','RTICAN','UnitType','MESSAGE','Identifier','TX','DialogType','MSVC','BlockSet','RTICAN','SlaveProcessor','CAN'))  RTIBlockInterface=struct('InputPortsWidth',int32([1 1 1 1]),'InputPortsActive',[1 1 1 1],'InputPortsName',{{'ACC_ObjLatPos','ACC_ObjDist','ACC_ObjRelSpd','ACC_ObjStatus'}},'InputPortsDataType',{{'SS_DOUBLE','SS_DOUBLE','SS_DOUBLE','SS_DOUBLE'}},'OutputPortsWidth',int32(0),'OutputPortsActive',0,'OutputPortsName',{{''}},'DialogFcn','rtican_message_interface_gui','BlockDisplay',{{'','center'}},'IconTransparency','on','InitLevel',3,'BlockName',struct('Token',{{'L_SCC2'}}),'SampleTime',{{0.02}},'TriggerPort',{{'none'}},'EnablePort',{{'none'}})  RTIBlockParameters=struct('BoardTypeNo',{{1,'OFF',[]}},'BoardNo',{{1,'ON',[1 16]}},'ChannelNo',{{1,'ON',[1 2]}},'Parameters',{{struct('DataFileSupport',struct('DataFileSelectedMaster',1,'DataFileSelectedLocal',1,'DataFileName',['c:\users\mpc\dropbox\hyundai car setup\hmc_can_for_ucb_v1.dbc|c:\users\mpc\dropbox\hyundai car setup\mobileye spec new\mobileye_mando_camera_ucb_v2.dbc|'],'DataFileDate',['26-Nov-2014 10:54:28'],'SelectedFile','c:\users\mpc_car\documents\github\mpc-car\dbcfiles\hmc_can_for_ucb_v2.dbc','InterfaceFcn','rtican_dbc_file_parser'),'Options',struct('StatusSelected',0,'TimeSelected',0,'DeltaTimeSelected',0,'DelayTimeSelected',0,'DelayTimeTXCommandSelected',0,'EncodeSetUnusedBitsToOne',0,'EnableMsgLoopback',0,'TriggerPort',struct('Selected',0,'TriggerType',0),'EnablePortSelected',0,'SignalOnPortnameSelected',1,'UserCoding',struct('Selected',0,'InterfaceFile','UserEncodingFile','FcnName','UserEncodeFcn','InportSelected',0,'InportWidth',1,'OutportSelected',0,'OutportWidth',1),'TerminationMsg',struct('Selected',0,'Byte0_7','0'),'InitialMsg',struct('Selected',0,'Byte0_7','0')),'Message',struct('MsgOnBlocknameSelected',1,'MsgName','L_SCC2','MsgIdFormat',0,'MsgId',257,'MsgLength',8,'NumSignals',4,'SampleTime',0.02,'StartTime',struct('Selected',0,'Value',0),'AutoRepeatTime',struct('Selected',0,'Value',0.1),'Timeout',struct('Selected',0,'Value',0.1),'DelayTime',struct('Selected',0,'Value',0.1),'Signal',struct('SgnName',{'ACC_ObjLatPos','ACC_ObjDist','ACC_ObjRelSpd','ACC_ObjStatus'},'SgnStartBit',{0,16,32,48},'SgnLength',{9,11,12,2},'ByteLayout',{0,0,0,0},'Factor',{0.1,0.1,0.1,1},'Offset',{-20,0,-170,0},'SgnComment',{'','','',''},'SgnUnit',{'m','m','m/s',''},'Min',{-20,0,-170,0},'Max',{31.1,204.7,239.5,3},'SgnType',{0,0,0,0},'SLDataType',{'SS_DOUBLE','SS_DOUBLE','SS_DOUBLE','SS_DOUBLE'},'DataType',{0,0,0,0},'ModeValue',{-1,-1,-1,-1}),'MsgIdNumFormat',0,'MsgComment',{{''}}),'Version',1.2,'general',struct('isFromLib',0)),'OFF',[]}},'GroupId',{{struct('Group',{{'RTICAN'}},'No',1,'Behavior',{{'NAMECHANGE'}},'BlockType',{{'SINK'}},'NameChangeFlag',0),'OFF',[]}},'SFcnRTICANMessage',{{struct('MsgType','TX','SFcnPortType','Scalar','MsgName','L_SCC2','MsgIdFormat','STD','MsgId',257,'MsgLength',8,'NumSignals',4,'SampleTime',0.02,'StartTime',struct('Selected','no','Value',0),'AutoRepeatTime',struct('Selected','no','Value',0.1),'Timeout',struct('Selected','no','Value',0.1),'Signal',struct('SgnName',{'ACC_ObjLatPos','ACC_ObjDist','ACC_ObjRelSpd','ACC_ObjStatus'},'SgnStartBit',{0,16,32,48},'SgnLength',{9,11,12,2},'ByteLayout',{['little endian'],['little endian'],['little endian'],['little endian']},'Factor',{0.1,0.1,0.1,1},'Offset',{-20,0,-170,0},'SgnType',{'standard','standard','standard','standard'},'SLDataType',{'SS_DOUBLE','SS_DOUBLE','SS_DOUBLE','SS_DOUBLE'},'DataType',{['unsigned int'],['unsigned int'],['unsigned int'],['unsigned int']},'ModeValue',{-1,-1,-1,-1}),'StatusSelected','no','TimeSelected','no','DeltaTimeSelected','no','DelayTimeSelected','no','DelayTimeTXCommandSelected','no','EncodeSetUnusedBitsToOne','no','EnableMsgLoopback','no','TriggerPort',struct('Selected','no','TriggerType',0),'EnablePortSelected','no','UserCoding',struct('Selected','no','InterfaceFile','UserEncodingFile','FcnName','UserEncodeFcn','InportSelected','no','InportWidth',1,'OutportSelected','no','OutportWidth',1),'TerminationMsg',struct('Selected','no','Byte0','0x00','Byte1','0x00','Byte2','0x00','Byte3','0x00','Byte4','0x00','Byte5','0x00','Byte6','0x00','Byte7','0x00'),'InitialMsg',struct('Selected','no','Byte0','0x00','Byte1','0x00','Byte2','0x00','Byte3','0x00','Byte4','0x00','Byte5','0x00','Byte6','0x00','Byte7','0x00'),'BoardType','DS1','BoardNo',1,'ControllerNo',1),'OFF',[]}},'TLCFileName',{{'rtican_tx_message','OFF',[]}})  RTISFcnParameters=struct('SFcnRTICANMessage','struct','TLCFileName','char')  RTIBlockParaDefault=struct('BoardTypeNo',4302,'BoardNo',1,'ChannelNo',1,'Parameters',struct('DataFileSupport',struct('DataFileSelectedMaster',0,'DataFileSelectedLocal',0,'DataFileName','','DataFileDate','','SelectedFile',['<no file selected>']),'Options',struct('StatusSelected',1,'TimeSelected',1,'DeltaTimeSelected',1,'DelayTimeSelected',1,'DelayTimeTXCommandSelected',0,'EncodeSetUnusedBitsToOne',0,'EnableMsgLoopback',0,'TriggerPort',struct('Selected',0,'TriggerType','rising'),'EnablePortSelected',0,'SignalOnPortnameSelected',1,'UserCoding',struct('Selected',0,'InterfaceFile','UserEncodingFile','FcnName','UserEncodeFcn','InportSelected',0,'InportWidth',1,'OutportSelected',0,'OutportWidth',1),'TerminationMsg',struct('Selected',0,'Byte0_7','0'),'InitialMsg',struct('Selected',0,'Byte0_7','0')),'Message',struct('MsgOnBlocknameSelected',0,'MsgName',['TX Message'],'MsgIdFormat',0,'MsgId',100,'MsgLength',8,'NumSignals',1,'SampleTime',-1,'StartTime',struct('Selected',0,'Value',0),'AutoRepeatTime',struct('Selected',0,'Value',0.1),'Timeout',struct('Selected',0,'Value',0.1),'DelayTime',struct('Selected',0,'Value',0.1),'Signal',struct('SgnName',['TX signal'],'SgnStartBit',0,'SgnLength',8,'SgnType',0,'ModeValue',-1,'DataType',0,'SLDataType','SS_DOUBLE','ByteLayout',0,'Factor',1,'Offset',0,'Min',0,'Max',255,'SgnComment',{{}},'SgnUnit',''),'MsgIdNumFormat',0,'MsgComment',{{''}}),'Version',1.2,'general',struct('isFromLib',1)),'GroupId',struct('Group',{{'RTICAN'}},'No',1,'Behavior',{{'NAMECHANGE'}},'BlockType',{{'SINK'}},'NameChangeFlag',0),'SFcnRTICANMessage',struct('MsgType','TX','MsgName',['TX Message'],'MsgIdFormat','STD','MsgId',100,'MsgLength',2,'NumSignals',1,'SampleTime',-1,'StartTime',struct('Selected','no','Value',0),'AutoRepeatTime',struct('Selected','no','Value',0.1),'Timeout',struct('Selected','no','Value',0.1),'DelayTime',struct('Selected','no','Value',0.1),'Signal',struct('SgnName',['TX signal'],'SgnStartBit',0,'SgnLength',8,'SgnType','standard','ModeValue',-1,'DataType',['unsigned int'],'ByteLayout',['little endian'],'SLDataType','SS_DOUBLE','Factor',1,'Offset',0),'StatusSelected','yes','TimeSelected','yes','DeltaTimeSelected','yes','DelayTimeSelected','yes','EnablePortSelected','no','EnableMsgLoopback','no','DelayTimeTXCommandSelected','no','EncodeSetUnusedBitsToOne','no','UserCoding',struct('Selected','no','InterfaceFile','UserDecodingFile','FcnName','UserDecodeFcn','InportSelected','no','InportWidth',1,'OutportSelected','no','OutportWidth',1),'TerminationMsg',struct('Selected','no','Byte0','0x00','Byte1','0x00','Byte2','0x00','Byte3','0x00','Byte4','0x00','Byte5','0x00','Byte6','0x00','Byte7','0x00'),'InitialMsg',struct('Selected','no','Byte0','0x00','Byte1','0x00','Byte2','0x00','Byte3','0x00','Byte4','0x00','Byte5','0x00','Byte6','0x00','Byte7','0x00'),'TriggerPort',struct('Selected','no','TriggerType','rising'),'BoardType','DS4302','BoardNo',1,'ControllerNo',1,'SFcnPortType','Scalar'),'TLCFileName','rtican_tx_message')
      settings: AttributesFormatString=Group Id: RTICAN1\n
  ObjectValid : Constant  Value=0
  Objvalid : Constant  Value=0
  Rate Transition2 : RateTransition  Integrity=off  OutPortSampleTime=0.02
  RelSpd : Constant  Value=0
  SCC1 Processing : Subsystem
  SCC2 Processing : Subsystem
  SetSpeed : Constant  Value=100
  Switch : Switch  Threshold=0.5
  disable : Constant  Value=5
  state : Constant  Value=0
  tag scope: acc_state=global
  wires:
  Objvalid/1 -> SCC1 Processing/3(spObjValid)
  SetSpeed/1 -> SCC1 Processing/4(uiSetSpdKph)
  Headway/1 -> SCC1 Processing/5(uiHeadwayState)
  ObjectValid/1 -> SCC2 Processing/1(spObjValid)
  Clearance/1 -> SCC2 Processing/2(spClearance)
  RelSpd/1 -> SCC2 Processing/3(spRelSpdCalMps)
  aReq/1 -> SCC1 Processing/2(aReq)  "aReq"
  Switch/1 -> SCC1 Processing/1(SCCmmState)
  disable/1 -> Switch/1
  DriverOverride_flag/1 -> Switch/2
  SCC1 Processing/1(aReqMax_CAN) -> L_SCC1/1
  SCC1 Processing/2(MainModeACC_CAN) -> L_SCC1/2
  SCC1 Processing/3(AliveCounterACC_CAN) -> L_SCC1/3
  SCC1 Processing/4(aReqMin_CAN) -> L_SCC1/4
  SCC1 Processing/5(VSetDis_CAN) -> L_SCC1/5
  SCC1 Processing/6(SCCInfoDisplay_CAN) -> L_SCC1/6  "opSCCInfoDisplay"
  SCC1 Processing/7(ACCFailInfo_CAN) -> L_SCC1/7
  SCC1 Processing/8(ACCMode_CAN) -> L_SCC1/8
  SCC1 Processing/9(StopReq_CAN) -> L_SCC1/9
  SCC1 Processing/10(PreFill_CAN) -> L_SCC1/10
  SCC1 Processing/11(ObjValid_CAN) -> L_SCC1/11
  SCC1 Processing/12(TakeOverReq_CAN) -> L_SCC1/12  "opTakeOverReq"
  SCC1 Processing/13(TauGapSet_CAN) -> L_SCC1/13
  SCC1 Processing/14(DriverAlertDisplay_CAN) -> L_SCC1/14  "opDriverAlertDisplay"
  SCC2 Processing/1(ACC_ObjLatPos_CAN) -> L_SCC2/1
  SCC2 Processing/2(ACC_ObjDist_CAN) -> L_SCC2/2
  SCC2 Processing/3(ACC_ObjRelSpd_CAN) -> L_SCC2/3
  SCC2 Processing/4(ACC_ObjStatus_CAN) -> L_SCC2/4
  state/1 -> [acc_state]
  Rate Transition2/1 -> Switch/3
  [acc_state] -> Rate Transition2/1
